simulink model "cascaded_droop_vi"  (R2021b)
settings: Solver=ode23t  StartTime=0.0  StopTime=20  RelTol=1e-3
values from neighbouring files (symbols this model uses):
  Cf_1 = 16e-6    (= 1.6e-05)    [parameters.m]
  fn = 50    [parameters.m]
  G_int = c2d(tf([wv 0],[1 wv]),Ts/2,'tustin')    [parameters.m]
  G_LPFd2 = c2d(tf([k*wn 0],[1 k*wn wn^2]),Ts/2,'tustin')    [parameters.m]
  Ilim = In    [parameters.m]
  ki_u = kp_u/Ti_u    [parameters.m]
  Kic_1 = (Rf_1)/T_i    (= 640)    [parameters.m]
  kp = delta_f/delta_P    (= 0.002)    [parameters.m]
  kp_u = Cf*w_c    [parameters.m]
  Kpc_1 = Rf_1/(exp(Rf_1/Lf_1*Ts/2)-1)    [parameters.m]
  Lf_1 = 5.6e-3    (= 0.0056)    [parameters.m]
  Lg_1 = 1e-3    (= 0.001)    [parameters.m]
  Lv = kQ/wn    [parameters.m]
  Pr = 2000    [parameters.m]
  RCf_1 = 0    [parameters.m]
  Rf_1 = 0.1    [parameters.m]
  Rg_1 = 0.08    [parameters.m]
  Rv = kQ/10    [parameters.m]
  Ts = 1/fs    (= 0.0003125)    [parameters.m]
  Ts_sim = Ts/100    (= 3.125e-06)    [parameters.m]
  Vdc = 800*sf_v    [parameters.m]
  Vn = 181*sqrt(2)*sf_v    [parameters.m]
  wn = 2*pi*fn    (= 314.159265359)    [parameters.m]
undefined symbols (not defined in the file or in its folder): DiscIntNeverNeededParam, plecs
libraries: spsVoltageMeasurementLib x15, spsCurrentMeasurementLib x12, spsabctoAlphaBetaZeroLib x10, spsThreePhaseSeriesRLCBranchLib x8, eeGeneralControl x7, spsThreePhaseVIMeasurementLib x4, spsGroundLib x3, spsThreePhaseSourceLib x2, spsDCVoltageSourceLib x2, spsEdgeDetectorLib x2, spsTriangleGeneratorLib x2, spsThreePhaseBreakerLib x2
(part 1 of 2)
settings Model: Creator=Thanh Hung Mai  LastModifiedBy=Thanh Hung Mai
settings DebuggingCC: UnconnectedInputMsg=none  UnconnectedOutputMsg=none  UnconnectedLineMsg=none
settings ModelReferenceCC: EnableRefExpFcnMdlSchedulingChecks=off
settings RTWCC: DLArmComputeVersion=20.02.1

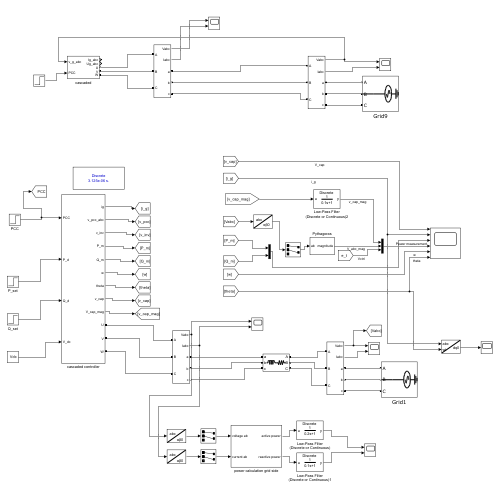
[thumbnail: Simulink's stored preview of the top-level diagram]
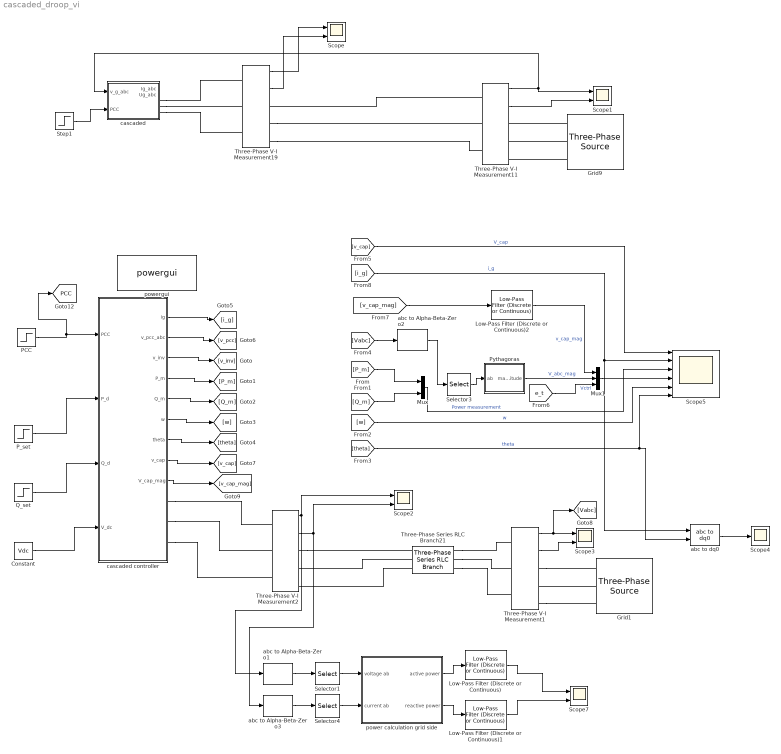
== system cascaded_droop_vi ==
  Constant : Constant  Value=Vdc
  Grid1 : spsThreePhaseSourceLib/Three-Phase Source  InternalConnection=Yg  VoltagePhases=off  Voltage=sqrt(3)*Vn/(sqrt(2))  PhaseAngle=20  Voltage_phases=[25e3 25e3 25e3]/sqrt(3)  PhaseAngles_phases=[0 -120 +120]  Frequency=50  NonIdealSource=off  SpecifyImpedance=off  Resistance=0  Inductance=0  ShortCircuitLevel=10e6  BaseVoltage=sqrt(3)*Vn/sqrt(2)  XRratio=2  BusType=swing  Pref=0  Qref=0  Prefabc=[10e3, 10e3, 10e3]  Qrefabc=[0, 0, 0]  Qmin=-inf  Qmax=inf
  Grid9 : spsThreePhaseSourceLib/Three-Phase Source  InternalConnection=Yg  VoltagePhases=off  Voltage=sqrt(3)*Vn/(sqrt(2))  PhaseAngle=0  Voltage_phases=[25e3 25e3 25e3]/sqrt(3)  PhaseAngles_phases=[0 -120 +120]  Frequency=fn  NonIdealSource=off  SpecifyImpedance=off  Resistance=0  Inductance=0  ShortCircuitLevel=10e6  BaseVoltage=sqrt(3)*Vn/sqrt(2)  XRratio=2  BusType=swing  Pref=0  Qref=0  Prefabc=[10e3, 10e3, 10e3]  Qrefabc=[0, 0, 0]  Qmin=-inf  Qmax=inf
  Low-Pass Filter (Discrete or Continuous) : eeGeneralControl/Low-Pass Filter (Discrete or Continuous)  K=1  T=0.2  B=inf  A=-inf  init_option=Inherited from block input  x0=0  Ts=-1
  Low-Pass Filter (Discrete or Continuous)1 : eeGeneralControl/Low-Pass Filter (Discrete or Continuous)  K=1  T=0.1  B=inf  A=-inf  init_option=Inherited from block input  x0=0  Ts=-1
  Low-Pass Filter (Discrete or Continuous)2 : eeGeneralControl/Low-Pass Filter (Discrete or Continuous)  K=1  T=0.1  B=inf  A=-inf  init_option=Inherited from block input  x0=0  Ts=-1
  Mux : Mux  Inputs=2
  Mux1 : Mux  Inputs=3
  PCC : Step  Time=0.4  SampleTime=Ts_sim
  P_set : Step  After=1000  SampleTime=Ts_sim
  Pythagoras : Subsystem
  Q_set : Step  Time=0  After=0  SampleTime=Ts_sim
  Scope{,1..3,7} (5 alike) : Scope  NumInputPorts=2
  Scope4 : Scope
  Scope5 : Scope  NumInputPorts=6
  Selector1 : Selector  IndexMode=Zero-based  InputPortWidth=3  IndexOptions=Index vector (dialog)  Indices=[0 1]  OutputSizes=1
  Selector3 : Selector  IndexMode=Zero-based  InputPortWidth=3  IndexOptions=Index vector (dialog)  Indices=[0 1]  OutputSizes=1
  Selector4 : Selector  IndexMode=Zero-based  InputPortWidth=3  IndexOptions=Index vector (dialog)  Indices=[0 1]  OutputSizes=1
  Step1 : Step  Time=0.5  SampleTime=0
  Three-Phase Series RLC Branch21 : spsThreePhaseSeriesRLCBranchLib/Three-Phase Series RLC Branch  LConnTagsString=A|B|C  RConnTagsString=A|B|C  BranchType=RL  Resistance=0.55  Inductance=4.39e-3  Capacitance=1e-6  Measurements=None
  Three-Phase V-I Measurement{1..2,11,19} (4 alike) : spsThreePhaseVIMeasurementLib/Three-Phase V-I Measurement  VoltageMeasurement=phase-to-ground  SetLabelV=off  LabelV=Vabc  Vpu=off  VpuLL=off  CurrentMeasurement=yes  SetLabelI=off  LabelI=Iabc  Ipu=off  Pbase=100e6  Vbase=500e3  OutputType=Complex  PhasorSimulation=off  PSBequivalent=0
  abc to Alpha-Beta-Zero1 : spsabctoAlphaBetaZeroLib/abc to Alpha-Beta-Zero
  abc to Alpha-Beta-Zero2 : spsabctoAlphaBetaZeroLib/abc to Alpha-Beta-Zero
  abc to Alpha-Beta-Zero3 : spsabctoAlphaBetaZeroLib/abc to Alpha-Beta-Zero
  abc to dq0 : spsabctodq0Lib/abc to dq0  Alignment=90 degrees behind phase A axis
  cascaded : Subsystem  VariantControl=cascaded
  cascaded controller : Subsystem  VariantControl=cascaded
  power calculation grid side : Subsystem
  powergui : spspowerguiLib/powergui  Priority=1  SimulationMode=Discrete  SampleTime=Ts_sim  frequency=60  Iterations=50  frequencyindice=50  Pbase=100e6  ErrMax=1e-4  UnitsV=kV  UnitsW=MW  buscounter=0  FunctionMessages=off  echomessages=off  EnableUseOfTLC=off  CurrentSourceSwitches=off  DisableSnubberDevices=off  DisableRonSwitches=off  DisableVfSwitches=off  DisplayEquations=off  AutomaticDiscreteSolvers=off  SolverType=Backward Euler  Interpol=off  ExternalGateDelay=off  methode=off  Ts=0  x0status=blocks  SPID=on  SwTol=0  HookPort=off  NonlinearTolerance=1e-4  nMaxIteration=100  ContinueOnMaxIteration=off  RestoreLinks=warning  ResistiveCurrentMeasurement=off  Frange=[0:2:500]  Ylog=off  Xlog=on  ShowGrid=off  save=off  variable=ZData  structure=0  ZoomFFT=off  StartTime=0.0  cycles=1  DisplayStyle=1  fundamental=60  FreqAxis=off  MaxFrequency=1000  frequencyindicesteady=1  RmsSteady=1  display=off
  tag scope: PCC=global
  wires:
  Three-Phase V-I Measurement11/1 -> cascaded/1(v_g_abc), Scope1/1
  Step1/1 -> cascaded/2(PCC)
  Three-Phase V-I Measurement19/1 -> Scope/1
  Three-Phase V-I Measurement19/2 -> Scope/2
  Three-Phase V-I Measurement11/2 -> Scope1/2
  [theta] -> abc to dq0/2, Scope5/6  "theta"
  cascaded controller/1(ig) -> [i_g]
  abc to Alpha-Beta-Zero1/1 -> Selector1/1
  [Q_m] -> Mux/2
  Q_set/1 -> cascaded controller/3(Q_d)
  Low-Pass Filter (Discrete or Continuous)/1 -> Scope7/1
  Selector1/1 -> power calculation grid side/1(voltage ab)
  Low-Pass Filter (Discrete or Continuous)1/1 -> Scope7/2
  cascaded controller/8(v_cap) -> [v_cap]
  Pythagoras/1(magnitude) -> Mux1/2  "V_abc_mag"
  Constant/1 -> cascaded controller/4(V_dc)
  [v_cap] -> Scope5/1  "V_cap"
  [P_m] -> Mux/1
  Three-Phase V-I Measurement2/1 -> abc to Alpha-Beta-Zero1/1, Scope2/1
  Three-Phase V-I Measurement2/2 -> abc to Alpha-Beta-Zero3/1, Scope2/2
  cascaded controller/9(V_cap_mag) -> [v_cap_mag]
  power calculation grid side/1(active power) -> Low-Pass Filter (Discrete or Continuous)/1
  Selector4/1 -> power calculation grid side/2(current ab)
  cascaded controller/6(w) -> [w]
  cascaded controller/4(P_m) -> [P_m]
  cascaded controller/3(v_inv) -> [v_inv]
  cascaded controller/7(theta) -> [theta]
  cascaded controller/5(Q_m) -> [Q_m]
  Low-Pass Filter (Discrete or Continuous)2/1 -> Mux1/1  "v_cap_mag"
  P_set/1 -> cascaded controller/2(P_d)
  [e_t] -> Mux1/3  "Vctrl"
  cascaded controller/2(v_pcc_abc) -> [v_pcc]
  PCC/1 -> [PCC], cascaded controller/1(PCC)
  abc to Alpha-Beta-Zero3/1 -> Selector4/1
  abc to Alpha-Beta-Zero2/1 -> Selector3/1
  Three-Phase V-I Measurement1/1 -> [Vabc], Scope3/1
  [Vabc] -> abc to Alpha-Beta-Zero2/1
  [w] -> Scope5/5  "w"
  Mux1/1 -> Scope5/4
  power calculation grid side/2(reactive power) -> Low-Pass Filter (Discrete or Continuous)1/1
  [i_g] -> abc to dq0/1, Scope5/2  "i_g"
  Selector3/1 -> Pythagoras/1(ab)
  [v_cap_mag] -> Low-Pass Filter (Discrete or Continuous)2/1
  Three-Phase V-I Measurement1/2 -> Scope3/2
  abc to dq0/1 -> Scope4/1
  Mux/1 -> Scope5/3  "Power measurement"
  connections:
  Three-Phase V-I Measurement11/LConn1 -- Three-Phase V-I Measurement19/RConn1
  cascaded/RConn3 -- Three-Phase V-I Measurement19/LConn3
  cascaded/RConn2 -- Three-Phase V-I Measurement19/LConn2
  Three-Phase V-I Measurement19/RConn3 -- Three-Phase V-I Measurement11/LConn3
  cascaded/RConn1 -- Three-Phase V-I Measurement19/LConn1
  Grid9/RConn1 -- Three-Phase V-I Measurement11/RConn1
  Three-Phase V-I Measurement19/RConn2 -- Three-Phase V-I Measurement11/LConn2
  Grid9/RConn2 -- Three-Phase V-I Measurement11/RConn2
  Grid9/RConn3 -- Three-Phase V-I Measurement11/RConn3
  Three-Phase V-I Measurement1/RConn1 -- Grid1/RConn1
  cascaded controller/RConn2 -- Three-Phase V-I Measurement2/LConn2
  Grid1/RConn2 -- Three-Phase V-I Measurement1/RConn2
  Three-Phase V-I Measurement1/RConn3 -- Grid1/RConn3
  cascaded controller/RConn1 -- Three-Phase V-I Measurement2/LConn1
  cascaded controller/RConn3 -- Three-Phase V-I Measurement2/LConn3
  Three-Phase V-I Measurement2/RConn1 -- Three-Phase Series RLC Branch21/RConn1
  Three-Phase Series RLC Branch21/RConn2 -- Three-Phase V-I Measurement2/RConn2
  Three-Phase Series RLC Branch21/RConn3 -- Three-Phase V-I Measurement2/RConn3
  Three-Phase Series RLC Branch21/LConn1 -- Three-Phase V-I Measurement1/LConn1
  Three-Phase Series RLC Branch21/LConn2 -- Three-Phase V-I Measurement1/LConn2
  Three-Phase Series RLC Branch21/LConn3 -- Three-Phase V-I Measurement1/LConn3

== system cascaded_droop_vi/Pythagoras ==
  ab : Inport
  Sqrt : Sqrt  SaturateOnIntegerOverflow=on
  Square : Math  Operator=square  SignedPower=on  RndMeth=Zero  SaturateOnIntegerOverflow=on
  Sum of Elements : Sum  Inputs=+
  magnitude : Outport  VectorParamsAs1DForOutWhenUnconnected=off
  wires:
  Sqrt/1 -> magnitude/1
  ab/1 -> Square/1
  Square/1 -> Sum of Elements/1
  Sum of Elements/1 -> Sqrt/1

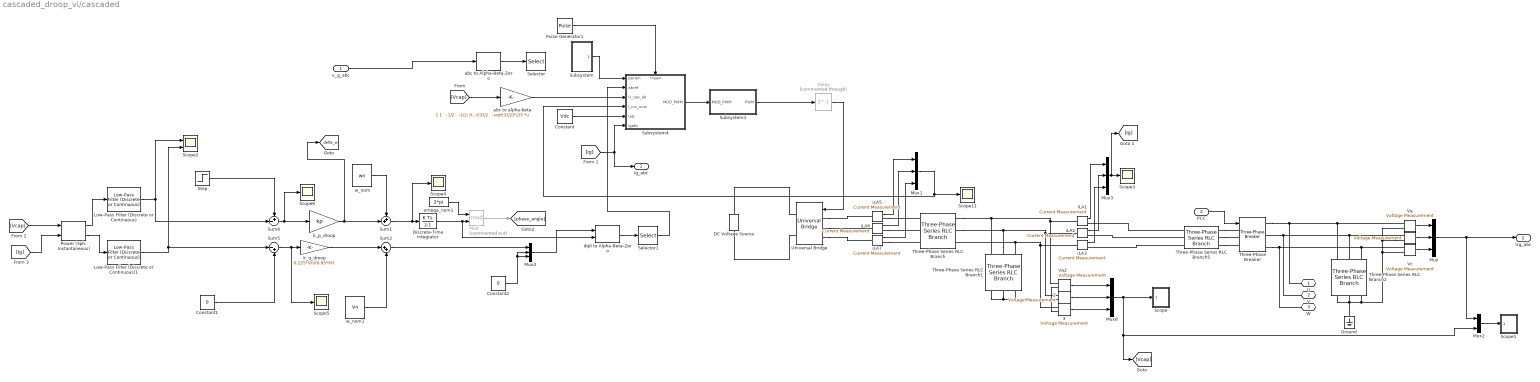
== system cascaded_droop_vi/cascaded ==
  v_g_abc : Inport
  PCC : Inport  Port=2
  "   " : spsVoltageMeasurementLib/Voltage Measurement  PhasorSimulation=off  OutputType=Complex  PSBequivalent=0
  "   2" : spsVoltageMeasurementLib/Voltage Measurement  PhasorSimulation=off  OutputType=Complex  PSBequivalent=0
  "   3" : spsVoltageMeasurementLib/Voltage Measurement  PhasorSimulation=off  OutputType=Complex  PSBequivalent=0
  Constant : Constant  Value=Vdc
  Constant1 : Constant  Value=0
  Constant2 : Constant  Value=0
  DC Voltage Source : spsDCVoltageSourceLib/DC Voltage Source  Amplitude=Vdc  Measurements=None
  Delay : Delay  Commented=through  DelayLength=1
  Discrete-Time Integrator : DiscreteIntegrator  SampleTime=-1  ICPrevOutput=DiscIntNeverNeededParam  ICPrevScaledInput=DiscIntNeverNeededParam
  Ground : spsGroundLib/Ground  LConnTagsString=a
  Low-Pass Filter (Discrete or Continuous) : eeGeneralControl/Low-Pass Filter (Discrete or Continuous)  K=1  T=0.2  B=inf  A=-inf  init_option=Inherited from block input  x0=0  Ts=-1
  Low-Pass Filter (Discrete or Continuous)1 : eeGeneralControl/Low-Pass Filter (Discrete or Continuous)  K=1  T=0.2  B=inf  A=-inf  init_option=Inherited from block input  x0=0  Ts=-1
  Mod : Math  Commented=on  Operator=mod  SaturateOnIntegerOverflow=on
  Mux{,1,3..4,8} (5 alike) : Mux  Inputs=3
  Mux2 : Mux  Inputs=2
  "Power (3ph, Instantaneous) " : spsPower3phInstantaneousLib/Power (3ph, Instantaneous)
  Pulse Generator1 : DiscretePulseGenerator  PulseType=Time based  Period=Ts/2%1/1.5e5  PulseWidth=50
  Scope : Subsystem  LoadFcn=plecs('sl', 300);  InitFcn=plecs('sl', 314);  StartFcn=plecs('sl', 308);  StopFcn=plecs('sl', 309);  mask{Settings=<binary blob, 1052 chars, not shown>}
      mask init:
      | plecs('sl', 315);
      settings: CopyFcn=plecs('sl', 303);  DeleteFcn=plecs('sl', 305);  UndoDeleteFcn=plecs('sl', 306);  PreSaveFcn=plecs('sl', 311);  NameChangeFcn=plecs('sl', 310);  DestroyFcn=plecs('sl', 307);  OpenFcn=plecs('sl', 302);  ErrorFcn=plerrorfcn
      mask Display: plot([0.1 0.9 0.9 0.1 0.1], [0.9 0.9 0.5 0.5 0.9])
  Scope1 : Subsystem  LoadFcn=plecs('sl', 300);  InitFcn=plecs('sl', 314);  StartFcn=plecs('sl', 308);  StopFcn=plecs('sl', 309);  mask{Settings=<binary blob, 1032 chars, not shown>}
      mask init:
      | plecs('sl', 315);
      settings: CopyFcn=plecs('sl', 303);  DeleteFcn=plecs('sl', 305);  UndoDeleteFcn=plecs('sl', 306);  PreSaveFcn=plecs('sl', 311);  NameChangeFcn=plecs('sl', 310);  DestroyFcn=plecs('sl', 307);  OpenFcn=plecs('sl', 302);  ErrorFcn=plerrorfcn
      mask Display: plot([0.1 0.9 0.9 0.1 0.1], [0.9 0.9 0.5 0.5 0.9])
  Scope{3..6,11} (5 alike) : Scope
  Scope2 : Scope  NumInputPorts=2
  Selector : Selector  IndexMode=Zero-based  InputPortWidth=3  IndexOptions=Index vector (dialog)  Indices=[0 1]  OutputSizes=1
  Selector1 : Selector  IndexMode=Zero-based  InputPortWidth=3  IndexOptions=Index vector (dialog)  Indices=[0 1]  OutputSizes=1
  Step : Step  After=Pr/2  SampleTime=0
  Subsystem : Subsystem
  Subsystem1 : Subsystem
  Subsystem4 : Subsystem
  Sum1 : Sum  Inputs=++|
  Sum2 : Sum  Inputs=|++
  Sum5 : Sum  Inputs=|-+
  Sum6 : Sum  Inputs=+-|
  Three-Phase Series RLC Branch : spsThreePhaseSeriesRLCBranchLib/Three-Phase Series RLC Branch  LConnTagsString=A|B|C  RConnTagsString=A|B|C  BranchType=RL  Resistance=Rf_1  Inductance=Lf_1  Capacitance=1e-6  Measurements=None
  Three-Phase Series RLC Branch1 : spsThreePhaseSeriesRLCBranchLib/Three-Phase Series RLC Branch  LConnTagsString=A|B|C  RConnTagsString=A|B|C  BranchType=RC  Resistance=RCf_1  Inductance=0.1e-3  Capacitance=Cf_1  Measurements=None
  Three-Phase Series RLC Branch2 : spsThreePhaseSeriesRLCBranchLib/Three-Phase Series RLC Branch  LConnTagsString=A|B|C  RConnTagsString=A|B|C  BranchType=R  Resistance=400e3  Inductance=0.1e-3  Capacitance=Cf_1  Measurements=None
  Three-Phase Series RLC Branch5 : spsThreePhaseSeriesRLCBranchLib/Three-Phase Series RLC Branch  LConnTagsString=A|B|C  RConnTagsString=A|B|C  BranchType=RL  Resistance=Rg_1  Inductance=Lg_1  Capacitance=1e-6  Measurements=None
  Three-Phase Breaker : spsThreePhaseBreakerLib/Three-Phase Breaker  InitialState=open  SwitchA=on  SwitchB=on  SwitchC=on  SwitchTimes=[0.1 0.9]  External=on  BreakerResistance=Ronb  SnubberResistance=Rsb  SnubberCapacitance=inf  Measurements=None
  Universal Bridge : spsUniversalBridgeLib/Universal Bridge  Arms=3  SnubberResistance=Rsi  SnubberCapacitance=inf  Device=IGBT / Diodes  Ron=Roni  Lon=0  ForwardVoltages="[  0  0  ]"  ForwardVoltage=0  GTOparameters=[ 10e-6 , 20e-6 ]  IGBTparameters=[ 1e-6 , 2e-6 ]  Measurements=None  Measurements_2=None  converterType=Rectifier
  Va : spsVoltageMeasurementLib/Voltage Measurement  PhasorSimulation=off  OutputType=Complex  PSBequivalent=0
  Va2 : spsVoltageMeasurementLib/Voltage Measurement  PhasorSimulation=off  OutputType=Complex  PSBequivalent=0
  Vc : spsVoltageMeasurementLib/Voltage Measurement  PhasorSimulation=off  OutputType=Complex  PSBequivalent=0
  abc to Alpha-Beta-Zero : spsabctoAlphaBetaZeroLib/abc to Alpha-Beta-Zero
  abc to alpha-beta : Gain  Gain="[ 1   -1/2   -1/2; 0   sqrt(3)/2   -sqrt(3)/2]*2/3"  Multiplication=Matrix(K*u) (u vector)  SaturateOnIntegerOverflow=on  OutDataTypeStr=Inherit: Same as input  ParamDataTypeStr=Inherit: Same as input
  dq0 to Alpha-Beta-Zero : spsdq0toAlphaBetaZeroLib/dq0 to Alpha-Beta-Zero  Alignment=90 degrees behind phase A axis
  iLA{1..3,5..7} (6 alike) : spsCurrentMeasurementLib/Current Measurement  PhasorSimulation=off  OutputType=Complex  PSBequivalent=0
  k_p_droop : Gain  Gain=kp
  k_q_droop : Gain  Gain=0.225*Vn/(0.95*Pr)
  omega_nom1 : Constant  Value=2*pi
  w_nom : Constant  Value=wn
  w_nom1 : Constant  Value=Vn
  U : PMIOPort  Side=Right
  V : PMIOPort  Port=2  Side=Right
  W : PMIOPort  Port=3  Side=Right
  Ig_abc : Outport  VectorParamsAs1DForOutWhenUnconnected=off
  Ug_abc : Outport  Port=2  VectorParamsAs1DForOutWhenUnconnected=off
  tag scope: delta_w=global
  wires:
  Mux2/1 -> Scope1/1(1)
  Subsystem4/1(MOD_PWM) -> Subsystem1/1(MOD_PWM)
  Mux/1 -> Mux2/1, Ug_abc/1
  Va2/1 -> Mux8/1
  iLA6/1 -> Mux1/2
  Constant/1 -> Subsystem4/5(Udc)
  Subsystem/1(param) -> Subsystem4/1(param)
  iLA3/1 -> Mux3/3
  PCC/1 -> Three-Phase Breaker/1
  Va/1 -> Mux/1
  Mux8/1 -> [Vcap], Mux2/2, Scope/1(1)
  Pulse Generator1/1 -> Subsystem4/Trigger
  iLA5/1 -> Mux1/1
  iLA2/1 -> Mux3/2
  iLA7/1 -> Mux1/3
  "   3"/1 -> Mux8/3
  "   "/1 -> Mux/2
  Mux1/1 -> Scope11/1, Subsystem4/4(I_inv_uvw)
  "   2"/1 -> Mux8/2
  Vc/1 -> Mux/3
  iLA1/1 -> Mux3/1
  Mux3/1 -> [Ig], Scope3/1
  Subsystem1/1(PWM) -> Delay/1
  Delay/1 -> Universal Bridge/1
  [Vcap] -> abc to alpha-beta/1
  [Ig] -> Ig_abc/1, Subsystem4/6(Igabc)
  [Vcap] -> "Power (3ph, Instantaneous) "/1
  [Ig] -> "Power (3ph, Instantaneous) "/2
  "Power (3ph, Instantaneous) "/1 -> Low-Pass Filter (Discrete or Continuous)/1
  "Power (3ph, Instantaneous) "/2 -> Low-Pass Filter (Discrete or Continuous)1/1
  Sum5/1 -> Scope5/1, k_q_droop/1
  w_nom1/1 -> Sum2/2
  Constant1/1 -> Sum5/2
  Sum6/1 -> Scope6/1, k_p_droop/1
  Step/1 -> Sum6/1
  w_nom/1 -> Sum1/1
  Sum2/1 -> Mux4/1
  Low-Pass Filter (Discrete or Continuous)/1 -> Sum6/2, Scope2/1
  Low-Pass Filter (Discrete or Continuous)1/1 -> Sum5/1, Scope2/2
  k_p_droop/1 -> [delta_w], Sum1/2
  Sum1/1 -> Scope4/1, Discrete-Time Integrator/1
  k_q_droop/1 -> Sum2/1
  Discrete-Time Integrator/1 -> dq0 to Alpha-Beta-Zero/2, Mod/2
  Mod/1 -> [phase_angle]
  omega_nom1/1 -> Mod/1
  abc to Alpha-Beta-Zero/1 -> Selector/1
  Mux4/1 -> dq0 to Alpha-Beta-Zero/1
  Constant2/1 -> Mux4/2, Mux4/3
  dq0 to Alpha-Beta-Zero/1 -> Selector1/1
  v_g_abc/1 -> abc to Alpha-Beta-Zero/1
  abc to alpha-beta/1 -> Subsystem4/3(U_cap_ab)
  Selector1/1 -> Subsystem4/2(abref)
  connections:
  "   "/LConn2 -- Ground/LConn1 -- Three-Phase Series RLC Branch2/RConn1 -- Three-Phase Series RLC Branch2/RConn2 -- Three-Phase Series RLC Branch2/RConn3 -- Vc/LConn2 -- Va/LConn2
  Three-Phase Series RLC Branch5/LConn1 -- Three-Phase Breaker/LConn1
  Three-Phase Breaker/RConn1 -- Three-Phase Series RLC Branch2/LConn1 -- Va/LConn1 -- U/RConn1
  DC Voltage Source/RConn1 -- Universal Bridge/RConn1
  iLA7/RConn1 -- Three-Phase Series RLC Branch/LConn3
  Va2/LConn2 -- Three-Phase Series RLC Branch1/RConn1 -- Three-Phase Series RLC Branch1/RConn2 -- Three-Phase Series RLC Branch1/RConn3 -- "   3"/LConn2 -- "   2"/LConn2
  Universal Bridge/LConn2 -- iLA6/LConn1
  iLA5/RConn1 -- Three-Phase Series RLC Branch/LConn1
  Three-Phase Series RLC Branch1/LConn2 -- Three-Phase Series RLC Branch/RConn2 -- iLA2/LConn1 -- "   2"/LConn1
  Three-Phase Series RLC Branch5/RConn1 -- iLA1/RConn1
  iLA6/RConn1 -- Three-Phase Series RLC Branch/LConn2
  Universal Bridge/LConn3 -- iLA7/LConn1
  Three-Phase Series RLC Branch5/LConn3 -- Three-Phase Breaker/LConn3
  Three-Phase Series RLC Branch/RConn3 -- Three-Phase Series RLC Branch1/LConn3 -- iLA3/LConn1 -- "   3"/LConn1
  "   "/LConn1 -- Three-Phase Series RLC Branch2/LConn2 -- Three-Phase Breaker/RConn2 -- V/RConn1
  DC Voltage Source/LConn1 -- Universal Bridge/RConn2
  Universal Bridge/LConn1 -- iLA5/LConn1
  Three-Phase Series RLC Branch5/LConn2 -- Three-Phase Breaker/LConn2
  Three-Phase Series RLC Branch5/RConn3 -- iLA3/RConn1
  Three-Phase Series RLC Branch/RConn1 -- Three-Phase Series RLC Branch1/LConn1 -- iLA1/LConn1 -- Va2/LConn1
  Three-Phase Breaker/RConn3 -- Three-Phase Series RLC Branch2/LConn3 -- Vc/LConn1 -- W/RConn1
  Three-Phase Series RLC Branch5/RConn2 -- iLA2/RConn1

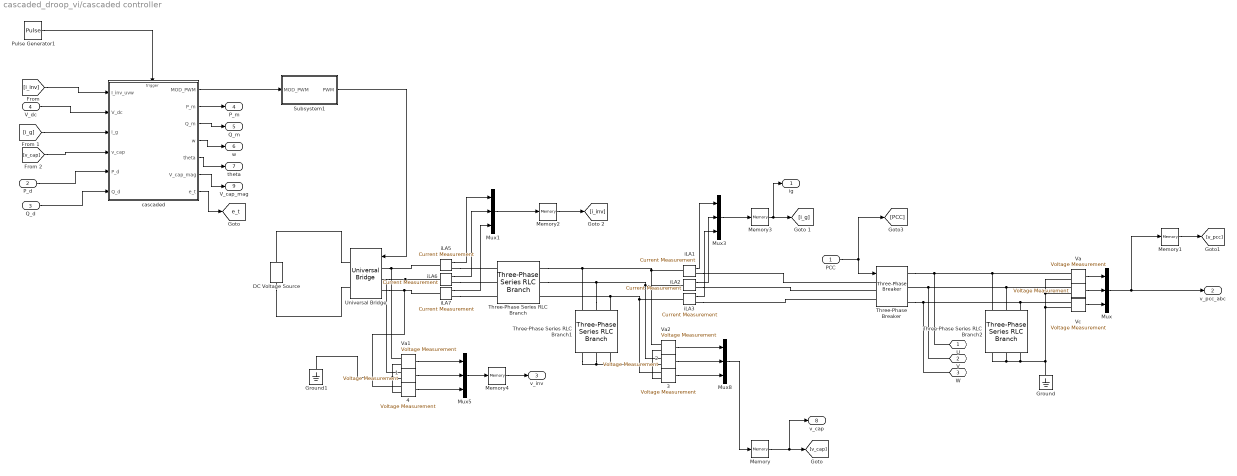
== system cascaded_droop_vi/cascaded controller ==
  PCC : Inport
  P_d : Inport  Port=2
  Q_d : Inport  Port=3
  V_dc : Inport  Port=4
     {,1..4} (5 alike) : spsVoltageMeasurementLib/Voltage Measurement  PhasorSimulation=off  OutputType=Complex  PSBequivalent=0
  DC Voltage Source : spsDCVoltageSourceLib/DC Voltage Source  Amplitude=Vdc  Measurements=None
  Ground : spsGroundLib/Ground  LConnTagsString=a
  Ground1 : spsGroundLib/Ground  LConnTagsString=a
  Memory{,1..4} (5 alike) : Memory
  Mux{,1,3,5,8} (5 alike) : Mux  Inputs=3
  Pulse Generator1 : DiscretePulseGenerator  PulseType=Time based  Period=Ts/2%1/1.5e5  PulseWidth=50
  Subsystem1 : Subsystem
  Three-Phase Series RLC Branch : spsThreePhaseSeriesRLCBranchLib/Three-Phase Series RLC Branch  LConnTagsString=A|B|C  RConnTagsString=A|B|C  BranchType=RL  Resistance=Rf_1  Inductance=Lf_1  Capacitance=1e-6  Measurements=None
  Three-Phase Series RLC Branch1 : spsThreePhaseSeriesRLCBranchLib/Three-Phase Series RLC Branch  LConnTagsString=A|B|C  RConnTagsString=A|B|C  BranchType=RC  Resistance=RCf_1  Inductance=0.1e-3  Capacitance=Cf_1  Measurements=None
  Three-Phase Series RLC Branch2 : spsThreePhaseSeriesRLCBranchLib/Three-Phase Series RLC Branch  LConnTagsString=A|B|C  RConnTagsString=A|B|C  BranchType=R  Resistance=400e3  Inductance=0.1e-3  Capacitance=Cf_1  Measurements=None
  Three-Phase Breaker : spsThreePhaseBreakerLib/Three-Phase Breaker  InitialState=open  SwitchA=on  SwitchB=on  SwitchC=on  SwitchTimes=[0.1 0.9]  External=on  BreakerResistance=Ronb  SnubberResistance=Rsb  SnubberCapacitance=inf  Measurements=None
  Universal Bridge : spsUniversalBridgeLib/Universal Bridge  Arms=3  SnubberResistance=Rsi  SnubberCapacitance=inf  Device=IGBT / Diodes  Ron=Roni  Lon=0  ForwardVoltages="[  0  0  ]"  ForwardVoltage=0  GTOparameters=[ 10e-6 , 20e-6 ]  IGBTparameters=[ 1e-6 , 2e-6 ]  Measurements=None  Measurements_2=None  converterType=Rectifier
  Va : spsVoltageMeasurementLib/Voltage Measurement  PhasorSimulation=off  OutputType=Complex  PSBequivalent=0
  Va1 : spsVoltageMeasurementLib/Voltage Measurement  PhasorSimulation=off  OutputType=Complex  PSBequivalent=0
  Va2 : spsVoltageMeasurementLib/Voltage Measurement  PhasorSimulation=off  OutputType=Complex  PSBequivalent=0
  Vc : spsVoltageMeasurementLib/Voltage Measurement  PhasorSimulation=off  OutputType=Complex  PSBequivalent=0
  cascaded : Subsystem
  iLA{1..3,5..7} (6 alike) : spsCurrentMeasurementLib/Current Measurement  PhasorSimulation=off  OutputType=Complex  PSBequivalent=0
  U : PMIOPort  Side=Right
  V : PMIOPort  Port=2  Side=Right
  W : PMIOPort  Port=3  Side=Right
  ig : Outport  VectorParamsAs1DForOutWhenUnconnected=off
  v_pcc_abc : Outport  Port=2  VectorParamsAs1DForOutWhenUnconnected=off
  v_inv : Outport  Port=3  VectorParamsAs1DForOutWhenUnconnected=off
  P_m : Outport  Port=4
  Q_m : Outport  Port=5
  w : Outport  Port=6
  theta : Outport  Port=7
  v_cap : Outport  Port=8  VectorParamsAs1DForOutWhenUnconnected=off
  V_cap_mag : Outport  Port=9  VectorParamsAs1DForOutWhenUnconnected=off
  tag scope: e_t=global
  wires:
  cascaded/1(MOD_PWM) -> Subsystem1/1(MOD_PWM)
  Mux/1 -> Memory1/1, v_pcc_abc/1
  Va2/1 -> Mux8/1
  iLA6/1 -> Mux1/2
  V_dc/1 -> cascaded/2(V_dc)
  iLA3/1 -> Mux3/3
  PCC/1 -> [PCC], Three-Phase Breaker/1
  Va/1 -> Mux/1
  iLA5/1 -> Mux1/1
  iLA2/1 -> Mux3/2
  iLA7/1 -> Mux1/3
  "   3"/1 -> Mux8/3
  "   "/1 -> Mux/2
  "   2"/1 -> Mux8/2
  Vc/1 -> Mux/3
  iLA1/1 -> Mux3/1
  Mux3/1 -> Memory3/1
  Subsystem1/1(PWM) -> Universal Bridge/1
  [i_g] -> cascaded/3(i_g)
  "   4"/1 -> Mux5/3
  Va1/1 -> Mux5/1
  "   1"/1 -> Mux5/2
  Memory/1 -> v_cap/1, [v_cap]
  Memory1/1 -> [v_pcc]
  Mux1/1 -> Memory2/1
  Memory2/1 -> [i_inv]
  [i_inv] -> cascaded/1(I_inv_uvw)
  [v_cap] -> cascaded/4(v_cap)
  Memory3/1 -> ig/1, [i_g]
  Mux5/1 -> Memory4/1
  Memory4/1 -> v_inv/1
  cascaded/5(theta) -> theta/1
  cascaded/4(w) -> w/1
  cascaded/3(Q_m) -> Q_m/1
  cascaded/2(P_m) -> P_m/1
  Q_d/1 -> cascaded/6(Q_d)
  P_d/1 -> cascaded/5(P_d)
  cascaded/6(V_cap_mag) -> V_cap_mag/1
  Mux8/1 -> Memory/1
  cascaded/7(e_t) -> [e_t]
  Pulse Generator1/1 -> cascaded/Trigger
  connections:
  Three-Phase Series RLC Branch2/RConn2 -- "   "/LConn2 -- Va/LConn2 -- Vc/LConn2 -- Ground/LConn1 -- Three-Phase Series RLC Branch2/RConn3 -- Three-Phase Series RLC Branch2/RConn1
  iLA1/RConn1 -- Three-Phase Breaker/LConn1
  Three-Phase Breaker/RConn1 -- U/RConn1 -- Three-Phase Series RLC Branch2/LConn1 -- Va/LConn1
  DC Voltage Source/RConn1 -- Universal Bridge/RConn1
  iLA7/RConn1 -- Three-Phase Series RLC Branch/LConn3
  Va2/LConn2 -- Three-Phase Series RLC Branch1/RConn1 -- Three-Phase Series RLC Branch1/RConn2 -- Three-Phase Series RLC Branch1/RConn3 -- "   3"/LConn2 -- "   2"/LConn2
  Universal Bridge/LConn2 -- "   1"/LConn1 -- iLA6/LConn1
  iLA5/RConn1 -- Three-Phase Series RLC Branch/LConn1
  Three-Phase Series RLC Branch1/LConn2 -- Three-Phase Series RLC Branch/RConn2 -- iLA2/LConn1 -- "   2"/LConn1
  iLA6/RConn1 -- Three-Phase Series RLC Branch/LConn2
  Universal Bridge/LConn3 -- "   4"/LConn1 -- iLA7/LConn1
  iLA3/RConn1 -- Three-Phase Breaker/LConn3
  Three-Phase Series RLC Branch/RConn3 -- Three-Phase Series RLC Branch1/LConn3 -- iLA3/LConn1 -- "   3"/LConn1
  "   "/LConn1 -- Three-Phase Series RLC Branch2/LConn2 -- V/RConn1 -- Three-Phase Breaker/RConn2
  DC Voltage Source/LConn1 -- Universal Bridge/RConn2
  Universal Bridge/LConn1 -- Va1/LConn1 -- iLA5/LConn1
  iLA2/RConn1 -- Three-Phase Breaker/LConn2
  Three-Phase Series RLC Branch/RConn1 -- Three-Phase Series RLC Branch1/LConn1 -- iLA1/LConn1 -- Va2/LConn1
  Three-Phase Breaker/RConn3 -- Three-Phase Series RLC Branch2/LConn3 -- Vc/LConn1 -- W/RConn1
  Va1/LConn2 -- Ground1/LConn1 -- "   4"/LConn2 -- "   1"/LConn2

== system cascaded_droop_vi/power calculation grid side ==
  voltage ab : Inport
  current ab : Inport  Port=2
  Demux : Demux  Outputs=2
  Demux1 : Demux  Outputs=2
  Gain1 : Gain  Gain=3/2
  Gain3 : Gain  Gain=3/2
  Product{1,4..6} (4 alike) : Product  InputSameDT=on  SaturateOnIntegerOverflow=on  OutDataTypeStr=Inherit: Same as first input
  Sum2 : Sum  Inputs=+-
  Sum3 : Sum
  abc to alpha-beta3 : Subsystem
  active power : Outport
  reactive power : Outport  Port=2
  wires:
  Product6/1 -> Sum2/2
  Product1/1 -> Sum2/1
  Sum2/1 -> Gain1/1
  Gain3/1 -> active power/1
  Product5/1 -> Sum3/2
  Demux1/2 -> Product5/2, Product6/2
  Demux/2 -> Product5/1, Product1/1
  Product4/1 -> Sum3/1
  Demux1/1 -> Product4/2, Product1/2
  Demux/1 -> Product6/1, Product4/1
  Sum3/1 -> Gain3/1
  Gain1/1 -> reactive power/1
  current ab/1 -> Demux1/1
  voltage ab/1 -> Demux/1

== system cascaded_droop_vi/cascaded/Scope ==
  1 : Inport
  " 1 " : DataTypeConversion  SaturateOnIntegerOverflow=on  RndMeth=Zero
  " InputMux " : Mux  Inputs=1
  " S-Function " : S-Function  FunctionName=plecs  SFunctionDeploymentMode=off  EnableBusSupport=off
  wires:
  " 1 "/1 -> " InputMux "/1
  1/1 -> " 1 "/1
  " InputMux "/1 -> " S-Function "/1

== system cascaded_droop_vi/cascaded/Scope1 ==
  1 : Inport
  " 1 " : DataTypeConversion  SaturateOnIntegerOverflow=on  RndMeth=Zero
  " InputMux " : Mux  Inputs=1
  " S-Function " : S-Function  FunctionName=plecs  SFunctionDeploymentMode=off  EnableBusSupport=off
  wires:
  " InputMux "/1 -> " S-Function "/1
  1/1 -> " 1 "/1
  " 1 "/1 -> " InputMux "/1

== system cascaded_droop_vi/cascaded/Subsystem ==
  1/kp_i : Constant  Value=1/Kpc_1
  1/kp_u : Constant  Value=1/kp_u
  Bus Creator : BusCreator  Inputs=11
  E1 : Constant  Value=wn*Lf_1
  E2 : Constant  Value=Cf_1*wn
  Isat : Constant  Value=Ilim
  g_ff_i : Constant
  g_ff_v : Constant
  ki_i*Ts/2 : Constant  Value=Kic_1
  ki_u*Ts/2 : Constant  Value=ki_u
  kp_i : Constant  Value=Kpc_1
  kp_u : Constant  Value=kp_u
  param : Outport  VectorParamsAs1DForOutWhenUnconnected=off
  wires:
  Bus Creator/1 -> param/1
  g_ff_v/1 -> Bus Creator/11  "g_ff_v"
  g_ff_i/1 -> Bus Creator/10  "g_ff_i"
  Isat/1 -> Bus Creator/9  "Isat"
  E2/1 -> Bus Creator/8  "E2"
  1/kp_u/1 -> Bus Creator/7  "1/kp_u"
  ki_u*Ts/2/1 -> Bus Creator/6  "ki_u"
  kp_u/1 -> Bus Creator/5  "kp_u"
  E1/1 -> Bus Creator/4  "E1"
  1/kp_i/1 -> Bus Creator/3  "1/kp_i"
  ki_i*Ts/2/1 -> Bus Creator/2  "ki_i"
  kp_i/1 -> Bus Creator/1  "kp_i"

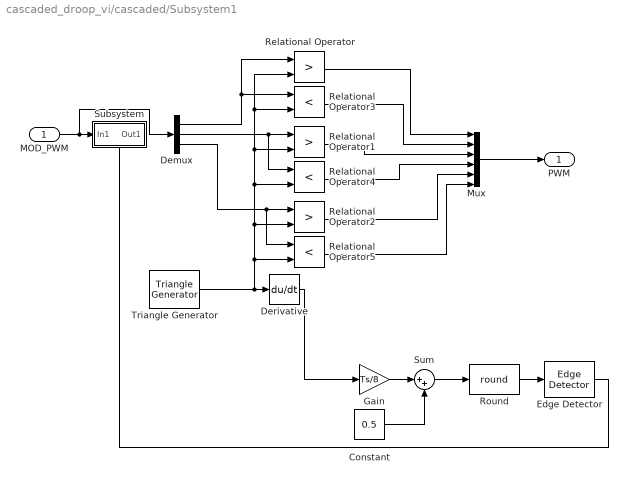
== system cascaded_droop_vi/cascaded/Subsystem1 ==
  MOD_PWM : Inport
  Constant : Constant  Value=0.5
  Demux : Demux  Outputs=3
  Derivative : Derivative
  Edge Detector : spsEdgeDetectorLib/Edge Detector  model=Either  ic=0  Ts=0
  Gain : Gain  Gain=Ts/8
  Mux : Mux  Inputs=6
  Relational Operator : RelationalOperator  Operator=>  OutDataTypeStr=boolean  RndMeth=Simplest
  Relational Operator1 : RelationalOperator  Operator=>  OutDataTypeStr=boolean  RndMeth=Simplest
  Relational Operator2 : RelationalOperator  Operator=>  OutDataTypeStr=boolean  RndMeth=Simplest
  Relational Operator3 : RelationalOperator  Operator=<  OutDataTypeStr=boolean  RndMeth=Simplest
  Relational Operator4 : RelationalOperator  Operator=<  OutDataTypeStr=boolean  RndMeth=Simplest
  Relational Operator5 : RelationalOperator  Operator=<  OutDataTypeStr=boolean  RndMeth=Simplest
  Round : Rounding  Operator=round
  Subsystem : Subsystem
  Sum : Sum  Inputs=|++
  Triangle Generator : spsTriangleGeneratorLib/Triangle Generator  Freq=fs  Phase=0  Ts=0
  PWM : Outport  VectorParamsAs1DForOutWhenUnconnected=off
  wires:
  Derivative/1 -> Gain/1
  Round/1 -> Edge Detector/1
  Sum/1 -> Round/1
  Constant/1 -> Sum/2
  Gain/1 -> Sum/1
  Relational Operator5/1 -> Mux/6
  Relational Operator2/1 -> Mux/5
  Relational Operator4/1 -> Mux/4
  Relational Operator1/1 -> Mux/3
  Relational Operator3/1 -> Mux/2
  Relational Operator/1 -> Mux/1
  Demux/3 -> Relational Operator2/1, Relational Operator5/1
  Demux/2 -> Relational Operator1/1, Relational Operator4/1
  Mux/1 -> PWM/1
  Demux/1 -> Relational Operator/1, Relational Operator3/1
  Triangle Generator/1 -> Relational Operator/2, Relational Operator3/2, Relational Operator1/2, Relational Operator4/2, Relational Operator2/2, Relational Operator5/2, Derivative/1
  Edge Detector/1 -> Subsystem/Trigger
  MOD_PWM/1 -> Demux/1, Subsystem/1(In1)

== system cascaded_droop_vi/cascaded/Subsystem4 ==
  param : Inport
  abref : Inport  Port=2
  U_cap_ab : Inport  Port=3
  I_inv_uvw : Inport  Port=4
  Udc : Inport  Port=5
  Igabc : Inport  Port=6
  Trigger : TriggerPort  VariantControl=Variant  PortDimensions=1
  Constant : Constant  Value=-2/9
  Subtract1 : Sum  Inputs=+-
  THI : Subsystem
  Virtual impedance1 : Subsystem
  abc to alpha-beta1 : Gain  Gain="[ 1   -1/2   -1/2; 0   sqrt(3)/2   -sqrt(3)/2]*2/3"  Multiplication=Matrix(K*u) (u vector)  SaturateOnIntegerOverflow=on  OutDataTypeStr=Inherit: Same as input  ParamDataTypeStr=Inherit: Same as input
  abc to alpha-beta2 : Gain  Gain="[ 1   -1/2   -1/2; 0   sqrt(3)/2   -sqrt(3)/2]*2/3"  Multiplication=Matrix(K*u) (u vector)  SaturateOnIntegerOverflow=on  OutDataTypeStr=Inherit: Same as input  ParamDataTypeStr=Inherit: Same as input
  alpha-beta to abc : Gain  Gain="[ 1   0; -1/2  sqrt(3)/2; -1/2  -sqrt(3)/2]"  Multiplication=Matrix(K*u) (u vector)  SaturateOnIntegerOverflow=on  OutDataTypeStr=Inherit: Same as input  ParamDataTypeStr=Inherit: Same as input
  current : Subsystem  VariantControl=PR
  voltage : Subsystem  VariantControl=PR
  MOD_PWM : Outport  VectorParamsAs1DForOutWhenUnconnected=off
  wires:
  Subtract1/1 -> voltage/2(U_ab_ref)
  Virtual impedance1/1(U_Lv_ab) -> Subtract1/2
  abc to alpha-beta1/1 -> Virtual impedance1/1(Ig_ab), voltage/4(Ig_ab)
  Igabc/1 -> abc to alpha-beta1/1
  param/1 -> current/1(param), voltage/1(param)
  I_inv_uvw/1 -> abc to alpha-beta2/1
  Udc/1 -> current/5(Udc)
  Constant/1 -> THI/1(THI gain)
  alpha-beta to abc/1 -> THI/2(abc)
  THI/1(abc_out) -> MOD_PWM/1
  U_cap_ab/1 -> voltage/3(U_ab), current/4(U_ab)
  abref/1 -> Subtract1/1
  voltage/1(I_ab_ref) -> current/2(I_ab_ref)
  abc to alpha-beta2/1 -> current/3(I_ab)
  current/1(U_ab_inv) -> THI/3(ab), alpha-beta to abc/1

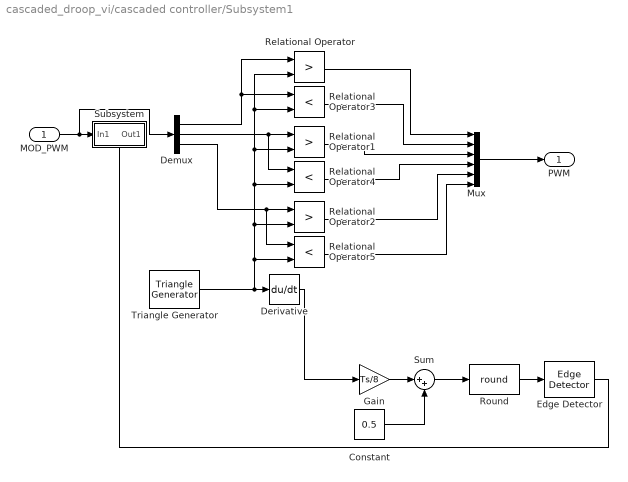
== system cascaded_droop_vi/cascaded controller/Subsystem1 ==
  MOD_PWM : Inport
  Constant : Constant  Value=0.5
  Demux : Demux  Outputs=3
  Derivative : Derivative
  Edge Detector : spsEdgeDetectorLib/Edge Detector  model=Either  ic=0  Ts=0
  Gain : Gain  Gain=Ts/8
  Mux : Mux  Inputs=6
  Relational Operator : RelationalOperator  Operator=>  OutDataTypeStr=boolean  RndMeth=Simplest
  Relational Operator1 : RelationalOperator  Operator=>  OutDataTypeStr=boolean  RndMeth=Simplest
  Relational Operator2 : RelationalOperator  Operator=>  OutDataTypeStr=boolean  RndMeth=Simplest
  Relational Operator3 : RelationalOperator  Operator=<  OutDataTypeStr=boolean  RndMeth=Simplest
  Relational Operator4 : RelationalOperator  Operator=<  OutDataTypeStr=boolean  RndMeth=Simplest
  Relational Operator5 : RelationalOperator  Operator=<  OutDataTypeStr=boolean  RndMeth=Simplest
  Round : Rounding  Operator=round
  Subsystem : Subsystem
  Sum : Sum  Inputs=|++
  Triangle Generator : spsTriangleGeneratorLib/Triangle Generator  Freq=fs  Phase=0  Ts=0
  PWM : Outport  VectorParamsAs1DForOutWhenUnconnected=off
  wires:
  Derivative/1 -> Gain/1
  Round/1 -> Edge Detector/1
  Sum/1 -> Round/1
  Constant/1 -> Sum/2
  Gain/1 -> Sum/1
  Relational Operator5/1 -> Mux/6
  Relational Operator2/1 -> Mux/5
  Relational Operator4/1 -> Mux/4
  Relational Operator1/1 -> Mux/3
  Relational Operator3/1 -> Mux/2
  Relational Operator/1 -> Mux/1
  Demux/3 -> Relational Operator2/1, Relational Operator5/1
  Demux/2 -> Relational Operator1/1, Relational Operator4/1
  Mux/1 -> PWM/1
  Demux/1 -> Relational Operator/1, Relational Operator3/1
  Triangle Generator/1 -> Relational Operator/2, Relational Operator3/2, Relational Operator1/2, Relational Operator4/2, Relational Operator2/2, Relational Operator5/2, Derivative/1
  Edge Detector/1 -> Subsystem/Trigger
  MOD_PWM/1 -> Demux/1, Subsystem/1(In1)

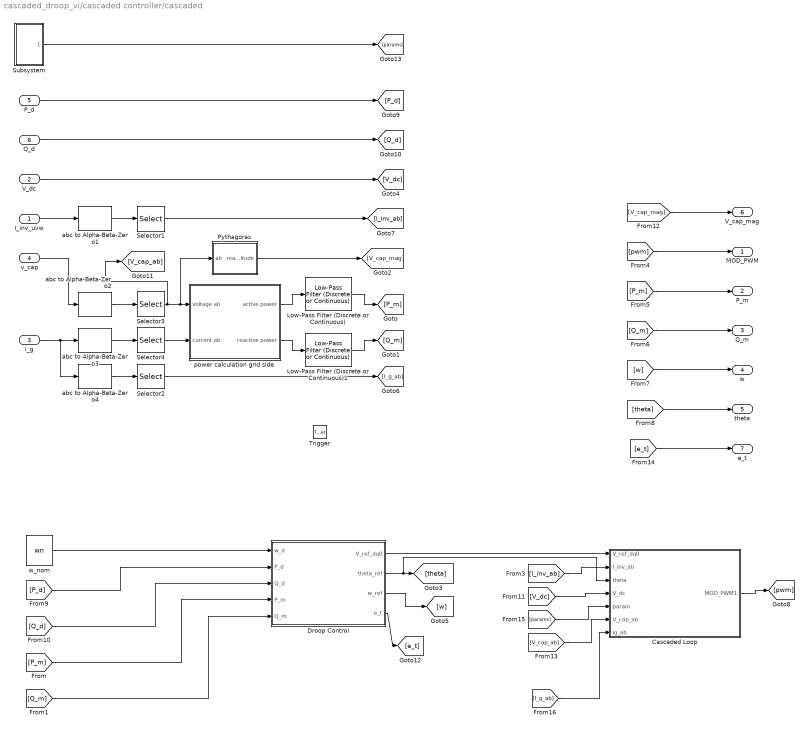
== system cascaded_droop_vi/cascaded controller/cascaded ==
  I_inv_uvw : Inport
  V_dc : Inport  Port=2
  i_g : Inport  Port=3
  v_cap : Inport  Port=4
  P_d : Inport  Port=5
  Q_d : Inport  Port=6
  Trigger : TriggerPort  VariantControl=(inherit)  PortDimensions=1
  Cascaded Loop : Subsystem
  Droop Control : Subsystem
  Low-Pass Filter (Discrete or Continuous) : eeGeneralControl/Low-Pass Filter (Discrete or Continuous)  K=1  T=0.1  B=inf  A=-inf  init_option=Inherited from block input  x0=0  Ts=-1
  Low-Pass Filter (Discrete or Continuous)1 : eeGeneralControl/Low-Pass Filter (Discrete or Continuous)  K=1  T=0.1  B=inf  A=-inf  init_option=Inherited from block input  x0=0  Ts=-1
  Pythagoras : Subsystem
  Selector{1..4} (4 alike) : Selector  IndexMode=Zero-based  InputPortWidth=3  IndexOptions=Index vector (dialog)  Indices=[0 1]  OutputSizes=1
  Subsystem : Subsystem
  abc to Alpha-Beta-Zero{1..4} (4 alike) : spsabctoAlphaBetaZeroLib/abc to Alpha-Beta-Zero
  power calculation grid side : Subsystem
  w_nom : Constant  Value=wn
  MOD_PWM : Outport  VectorParamsAs1DForOutWhenUnconnected=off
  P_m : Outport  Port=2  VectorParamsAs1DForOutWhenUnconnected=off
  Q_m : Outport  Port=3  VectorParamsAs1DForOutWhenUnconnected=off
  w : Outport  Port=4  VectorParamsAs1DForOutWhenUnconnected=off
  theta : Outport  Port=5  VectorParamsAs1DForOutWhenUnconnected=off
  V_cap_mag : Outport  Port=6  VectorParamsAs1DForOutWhenUnconnected=off
  e_t : Outport  Port=7  VectorParamsAs1DForOutWhenUnconnected=off
  wires:
  abc to Alpha-Beta-Zero2/1 -> Selector3/1
  v_cap/1 -> abc to Alpha-Beta-Zero2/1
  abc to Alpha-Beta-Zero3/1 -> Selector4/1
  i_g/1 -> abc to Alpha-Beta-Zero4/1, abc to Alpha-Beta-Zero3/1
  Pythagoras/1(magnitude) -> [V_cap_mag]
  w_nom/1 -> Droop Control/1(w_d)
  [P_d] -> Droop Control/2(P_d)
  [P_m] -> Droop Control/4(P_m)
  [Q_m] -> Droop Control/5(Q_m)
  [Q_d] -> Droop Control/3(Q_d)
  Droop Control/2(theta_ref) -> Cascaded Loop/3(theta), [theta]
  Droop Control/3(w_ref) -> [w]
  I_inv_uvw/1 -> abc to Alpha-Beta-Zero1/1
  abc to Alpha-Beta-Zero1/1 -> Selector1/1
  V_dc/1 -> [V_dc]
  abc to Alpha-Beta-Zero4/1 -> Selector2/1
  Selector2/1 -> [I_g_ab]
  [I_inv_ab] -> Cascaded Loop/2(I_inv_ab)
  Selector1/1 -> [I_inv_ab]
  Cascaded Loop/1(MOD_PWM1) -> [pwm]
  [pwm] -> MOD_PWM/1
  [P_m] -> P_m/1
  [Q_m] -> Q_m/1
  [w] -> w/1
  [theta] -> theta/1
  P_d/1 -> [P_d]
  Q_d/1 -> [Q_d]
  [V_dc] -> Cascaded Loop/4(V_dc)
  Selector3/1 -> [V_cap_ab], Pythagoras/1(ab), power calculation grid side/1(voltage ab)
  Selector4/1 -> power calculation grid side/2(current ab)
  power calculation grid side/1(active power) -> Low-Pass Filter (Discrete or Continuous)/1
  Low-Pass Filter (Discrete or Continuous)/1 -> [P_m]
  power calculation grid side/2(reactive power) -> Low-Pass Filter (Discrete or Continuous)1/1
  Low-Pass Filter (Discrete or Continuous)1/1 -> [Q_m]
  [V_cap_mag] -> V_cap_mag/1
  [V_cap_ab] -> Cascaded Loop/6(V_cap_ab)
  Droop Control/4(e_t) -> [e_t]
  [e_t] -> e_t/1
  Subsystem/1(param) -> [params]
  [params] -> Cascaded Loop/5(param)
  [I_g_ab] -> Cascaded Loop/7(ig_ab)
  Droop Control/1(V_ref_dq0) -> Cascaded Loop/1(V_ref_dq0)

== system cascaded_droop_vi/power calculation grid side/abc to alpha-beta3 ==
  abc : Inport
  Demux : Demux  Outputs=3
  Terminator1 : Terminator
  abc to Alpha-Beta-Zero : spsabctoAlphaBetaZeroLib/abc to Alpha-Beta-Zero
  alpha : Outport
  beta : Outport  Port=2
  wires:
  abc to Alpha-Beta-Zero/1 -> Demux/1
  abc/1 -> abc to Alpha-Beta-Zero/1
  Demux/3 -> Terminator1/1
  Demux/2 -> beta/1
  Demux/1 -> alpha/1

== system cascaded_droop_vi/cascaded/Subsystem1/Subsystem ==
  In1 : Inport
  Trigger : TriggerPort  VariantControl=Variant  PortDimensions=1
  Out1 : Outport  VectorParamsAs1DForOutWhenUnconnected=off
  wires:
  In1/1 -> Out1/1

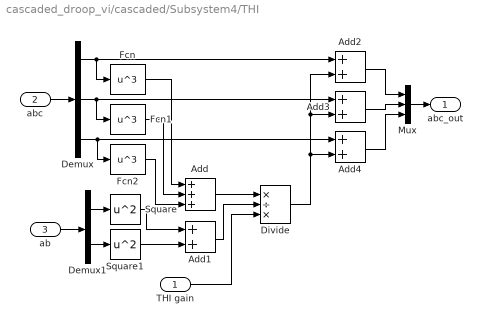
== system cascaded_droop_vi/cascaded/Subsystem4/THI ==
  THI gain : Inport
  abc : Inport  Port=2
  ab : Inport  Port=3
  Add : Sum  Inputs=+++
  Add{1..4} (4 alike) : Sum
  Demux : Demux  Outputs=3
  Demux1 : Demux  Outputs=2
  Divide : Product  Inputs=*/*
  Fcn : Fcn  Expr=u^3
  Fcn1 : Fcn  Expr=u^3
  Fcn2 : Fcn  Expr=u^3
  Mux : Mux  Inputs=3
  Square : Math  Operator=square  SignedPower=on  RndMeth=Zero  SaturateOnIntegerOverflow=on
  Square1 : Math  Operator=square  SignedPower=on  RndMeth=Zero  SaturateOnIntegerOverflow=on
  abc_out : Outport  VectorParamsAs1DForOutWhenUnconnected=off
  wires:
  Demux/2 -> Add3/1, Fcn1/1
  Fcn2/1 -> Add/3
  Fcn1/1 -> Add/2
  Fcn/1 -> Add/1
  Mux/1 -> abc_out/1
  Add4/1 -> Mux/3
  Add2/1 -> Mux/1
  Add3/1 -> Mux/2
  Divide/1 -> Add4/2, Add3/2, Add2/2
  THI gain/1 -> Divide/3
  Add1/1 -> Divide/2
  Add/1 -> Divide/1
  Square1/1 -> Add1/2
  Square/1 -> Add1/1
  Demux1/2 -> Square1/1
  Demux1/1 -> Square/1
  ab/1 -> Demux1/1
  Demux/1 -> Fcn/1, Add2/1
  Demux/3 -> Add4/1, Fcn2/1
  abc/1 -> Demux/1

== system cascaded_droop_vi/cascaded/Subsystem4/Virtual impedance1 ==
  Ig_ab : Inport
  Discrete Transfer Fcn2 : DiscreteTransferFcn  Numerator=G_int.num{1}  Denominator=G_int.den{1}
  Gain1 : Gain  Gain=Rv
  Gain2 : Gain  Gain=Lv
  Sum3 : Sum  Inputs=|++
  U_Lv_ab : Outport  VectorParamsAs1DForOutWhenUnconnected=off
  wires:
  Sum3/1 -> U_Lv_ab/1
  Gain1/1 -> Sum3/2
  Gain2/1 -> Sum3/1
  Ig_ab/1 -> Discrete Transfer Fcn2/1, Gain1/1
  Discrete Transfer Fcn2/1 -> Gain2/1

== system cascaded_droop_vi/cascaded/Subsystem4/current ==
  param : Inport
  I_ab_ref : Inport  Port=2
  I_ab : Inport  Port=3
  U_ab : Inport  Port=4
  Udc : Inport  Port=5
  Bus Selector : BusSelector  OutputSignals=E1,g_ff_v
  Delay : Delay  DelayLength=1  InitialCondition=0
  Discrete Transfer Fcn : DiscreteTransferFcn  Numerator=G_LPFd2.num{1}  Denominator=G_LPFd2.den{1}
  Divide : Product  Inputs=*/
  Gain : Gain  Gain=1/2
  Subtract : Sum  Inputs=+-
  Subtract1 : Sum  Inputs=+-
  Voltage_lim : Subsystem
  control_ab : Subsystem
  voltage_FF : Subsystem
  U_ab_inv : Outport  VectorParamsAs1DForOutWhenUnconnected=off
  wires:
  Discrete Transfer Fcn/1 -> voltage_FF/2(b)
  voltage_FF/1(ab_out) -> Voltage_lim/1(ab_in), Subtract/1
  Delay/1 -> control_ab/3(awr)
  Gain/1 -> Divide/2
  Divide/1 -> U_ab_inv/1
  Udc/1 -> Voltage_lim/2(Vdc), Gain/1
  U_ab/1 -> Discrete Transfer Fcn/1
  Subtract/1 -> Delay/1
  Bus Selector/2 -> voltage_FF/3(g_FF)  "<g_ff_v>"
  I_ab/1 -> Subtract1/2
  Subtract1/1 -> control_ab/1(in_ab)
  control_ab/1(out) -> voltage_FF/1(a)
  param/1 -> control_ab/2(param), Bus Selector/1
  I_ab_ref/1 -> Subtract1/1
  Voltage_lim/1(ab_out) -> Subtract/2, Divide/1

== system cascaded_droop_vi/cascaded/Subsystem4/voltage ==
  param : Inport
  U_ab_ref : Inport  Port=2
  U_ab : Inport  Port=3
  Ig_ab : Inport  Port=4
  Bus Selector : BusSelector  OutputSignals=g_ff_i,Isat
  Current_lim : Subsystem
  Delay : Delay  DelayLength=1  InitialCondition=0
  Subtract : Sum  Inputs=+-
  Subtract1 : Sum  Inputs=+-
  control_ab : Subsystem
  current_FF : Subsystem
  I_ab_ref : Outport  VectorParamsAs1DForOutWhenUnconnected=off
  wires:
  Bus Selector/2 -> Current_lim/2(Isat)  "<Isat>"
  U_ab_ref/1 -> Subtract1/1
  param/1 -> Bus Selector/1, control_ab/2(param)
  control_ab/1(out) -> current_FF/1(a)
  Subtract1/1 -> control_ab/1(in_ab)
  U_ab/1 -> Subtract1/2
  Bus Selector/1 -> current_FF/3(g_FF)  "<g_ff_i>"
  Subtract/1 -> Delay/1
  Ig_ab/1 -> current_FF/2(b)
  Current_lim/1(ab_out) -> I_ab_ref/1, Subtract/2
  Delay/1 -> control_ab/3(awr)
  current_FF/1(ab_out) -> Subtract/1, Current_lim/1(ab_in)

== system cascaded_droop_vi/cascaded controller/Subsystem1/Subsystem ==
  In1 : Inport
  Trigger : TriggerPort  VariantControl=Variant  PortDimensions=1
  Out1 : Outport  VectorParamsAs1DForOutWhenUnconnected=off
  wires:
  In1/1 -> Out1/1

== system cascaded_droop_vi/cascaded controller/cascaded/Cascaded Loop ==
  V_ref_dq0 : Inport
  I_inv_ab : Inport  Port=2
  theta : Inport  Port=3
  V_dc : Inport  Port=4
  param : Inport  Port=5
  V_cap_ab : Inport  Port=6
  ig_ab : Inport  Port=7
  Constant1 : Constant  Value=-2/9
  Scope : Scope
  Selector3 : Selector  IndexMode=Zero-based  InputPortWidth=3  IndexOptions=Index vector (dialog)  Indices=[0 1]  OutputSizes=1
  Subtract2 : Sum  Inputs=+-
  THI1 : Subsystem
  Virtual impedance : Subsystem
  alpha-beta to abc1 : Gain  Gain="[ 1   0; -1/2  sqrt(3)/2; -1/2  -sqrt(3)/2]"  Multiplication=Matrix(K*u) (u vector)  SaturateOnIntegerOverflow=on  OutDataTypeStr=Inherit: Same as input  ParamDataTypeStr=Inherit: Same as input
  current : Subsystem  VariantControl=PR
  dq0 to Alpha-Beta-Zero : spsdq0toAlphaBetaZeroLib/dq0 to Alpha-Beta-Zero  Alignment=90 degrees behind phase A axis
  voltage : Subsystem  VariantControl=PR
  MOD_PWM1 : Outport  VectorParamsAs1DForOutWhenUnconnected=off
  wires:
  dq0 to Alpha-Beta-Zero/1 -> Selector3/1
  V_ref_dq0/1 -> dq0 to Alpha-Beta-Zero/1
  Constant1/1 -> THI1/1(THI gain)
  THI1/1(abc_out) -> MOD_PWM1/1
  V_cap_ab/1 -> voltage/3(U_ab), current/4(U_ab)
  ig_ab/1 -> voltage/4(Ig_ab), Virtual impedance/1(Ig_ab)
  param/1 -> current/1(param), voltage/1(param)
  voltage/1(I_ab_ref) -> current/2(I_ab_ref)
  Subtract2/1 -> voltage/2(U_ab_ref)
  alpha-beta to abc1/1 -> THI1/2(abc)
  current/1(U_ab_inv) -> THI1/3(ab), alpha-beta to abc1/1
  Virtual impedance/1(U_Lv_ab) -> Subtract2/2
  V_dc/1 -> current/5(Udc)
  Selector3/1 -> Scope/1, Subtract2/1
  I_inv_ab/1 -> current/3(I_ab)
  theta/1 -> dq0 to Alpha-Beta-Zero/2

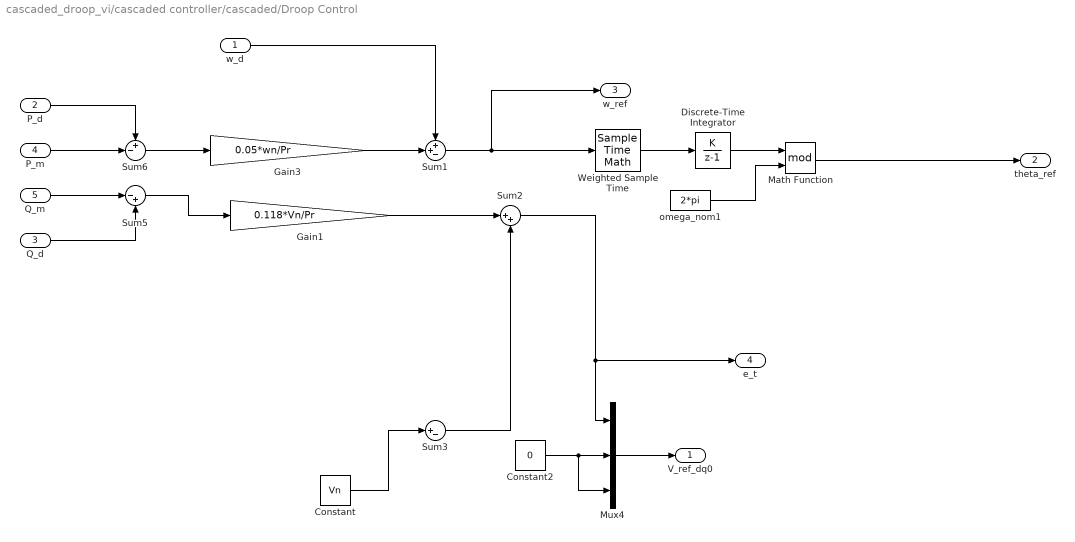
== system cascaded_droop_vi/cascaded controller/cascaded/Droop Control ==
  w_d : Inport
  P_d : Inport  Port=2
  Q_d : Inport  Port=3
  P_m : Inport  Port=4
  Q_m : Inport  Port=5
  Constant : Constant  Value=Vn
  Constant2 : Constant  Value=0
  Discrete-Time Integrator : DiscreteIntegrator  IntegratorMethod=Accumulation: Forward Euler  InitialCondition=pi*0  SampleTime=-1  ICPrevOutput=DiscIntNeverNeededParam  ICPrevScaledInput=DiscIntNeverNeededParam
  Gain1 : Gain  Gain=0.118*Vn/Pr
  Gain3 : Gain  Gain=0.05*wn/Pr
  Math Function : Math  Operator=mod  SignedPower=on  SaturateOnIntegerOverflow=on
  Mux4 : Mux  Inputs=3
  Sum1 : Sum  Inputs=++-
  Sum2 : Sum  Inputs=|++
  Sum3 : Sum  Inputs=|+-
  Sum5 : Sum  Inputs=|-+
  Sum6 : Sum  Inputs=+-|
  Weighted Sample Time : SampleTimeMath  TsampMathOp=*  TsampMathImp=Offline Scaling Adjustment
  omega_nom1 : Constant  Value=2*pi
  V_ref_dq0 : Outport
  theta_ref : Outport  Port=2
  w_ref : Outport  Port=3
  e_t : Outport  Port=4
  wires:
  Q_d/1 -> Sum5/2
  P_d/1 -> Sum6/1
  P_m/1 -> Sum6/2
  Q_m/1 -> Sum5/1
  Sum5/1 -> Gain1/1
  w_d/1 -> Sum1/1
  Sum3/1 -> Sum2/2
  Constant2/1 -> Mux4/3, Mux4/2
  Sum1/1 -> Weighted Sample Time/1, w_ref/1
  Mux4/1 -> V_ref_dq0/1
  Gain1/1 -> Sum2/1
  Constant/1 -> Sum3/1
  Sum2/1 -> Mux4/1, e_t/1
  Math Function/1 -> theta_ref/1
  omega_nom1/1 -> Math Function/2
  Discrete-Time Integrator/1 -> Math Function/1
  Weighted Sample Time/1 -> Discrete-Time Integrator/1
  Sum6/1 -> Gain3/1
  Gain3/1 -> Sum1/2

== system cascaded_droop_vi/cascaded controller/cascaded/Pythagoras ==
  ab : Inport
  Sqrt : Sqrt  SaturateOnIntegerOverflow=on
  Square : Math  Operator=square  SignedPower=on  RndMeth=Zero  SaturateOnIntegerOverflow=on
  Sum of Elements : Sum  Inputs=+
  magnitude : Outport  VectorParamsAs1DForOutWhenUnconnected=off
  wires:
  Sqrt/1 -> magnitude/1
  ab/1 -> Square/1
  Square/1 -> Sum of Elements/1
  Sum of Elements/1 -> Sqrt/1

== system cascaded_droop_vi/cascaded controller/cascaded/Subsystem ==
  1/kp_i : Constant  Value=1/Kpc_1
  1/kp_u : Constant  Value=1/kp_u
  Bus Creator : BusCreator  Inputs=11
  E1 : Constant  Value=wn*Lf_1
  E2 : Constant  Value=Cf_1*wn
  Isat : Constant  Value=Ilim
  g_ff_i : Constant
  g_ff_v : Constant
  ki_i*Ts/2 : Constant  Value=Kic_1
  ki_u*Ts/2 : Constant  Value=ki_u
  kp_i : Constant  Value=Kpc_1
  kp_u : Constant  Value=kp_u
  param : Outport  VectorParamsAs1DForOutWhenUnconnected=off
  wires:
  Bus Creator/1 -> param/1
  g_ff_v/1 -> Bus Creator/11  "g_ff_v"
  g_ff_i/1 -> Bus Creator/10  "g_ff_i"
  Isat/1 -> Bus Creator/9  "Isat"
  E2/1 -> Bus Creator/8  "E2"
  1/kp_u/1 -> Bus Creator/7  "1/kp_u"
  ki_u*Ts/2/1 -> Bus Creator/6  "ki_u"
  kp_u/1 -> Bus Creator/5  "kp_u"
  E1/1 -> Bus Creator/4  "E1"
  1/kp_i/1 -> Bus Creator/3  "1/kp_i"
  ki_i*Ts/2/1 -> Bus Creator/2  "ki_i"
  kp_i/1 -> Bus Creator/1  "kp_i"

== system cascaded_droop_vi/cascaded controller/cascaded/power calculation grid side ==
  voltage ab : Inport
  current ab : Inport  Port=2
  Demux : Demux  Outputs=2
  Demux1 : Demux  Outputs=2
  Gain1 : Gain  Gain=3/2
  Gain3 : Gain  Gain=3/2
  Product{1,4..6} (4 alike) : Product  InputSameDT=on  SaturateOnIntegerOverflow=on  OutDataTypeStr=Inherit: Same as first input
  Sum2 : Sum  Inputs=+-
  Sum3 : Sum
  abc to alpha-beta3 : Subsystem
  active power : Outport
  reactive power : Outport  Port=2
  wires:
  Product6/1 -> Sum2/2
  Product1/1 -> Sum2/1
  Sum2/1 -> Gain1/1
  Gain3/1 -> active power/1
  Product5/1 -> Sum3/2
  Demux1/2 -> Product5/2, Product6/2
  Demux/2 -> Product5/1, Product1/1
  Product4/1 -> Sum3/1
  Demux1/1 -> Product4/2, Product1/2
  Demux/1 -> Product6/1, Product4/1
  Sum3/1 -> Gain3/1
  Gain1/1 -> reactive power/1
  current ab/1 -> Demux1/1
  voltage ab/1 -> Demux/1

== system cascaded_droop_vi/cascaded/Subsystem4/current/Voltage_lim ==
  ab_in : Inport
  Vdc : Inport  Port=2
  Divide : Product  Inputs=*/
  Divide1 : Product  Inputs=**
  Gain : Gain  Gain=1/sqrt(3)
  Subsystem : Subsystem
  pythagoras : Subsystem
  ab_out : Outport  VectorParamsAs1DForOutWhenUnconnected=off
  wires:
  Gain/1 -> Divide/1, Subsystem/2(b)
  ab_in/1 -> Divide1/2, pythagoras/1(ab)
  pythagoras/1(|ab|) -> Subsystem/1(a)
  Vdc/1 -> Gain/1
  Subsystem/1(max) -> Divide/2
  Divide/1 -> Divide1/1
  Divide1/1 -> ab_out/1

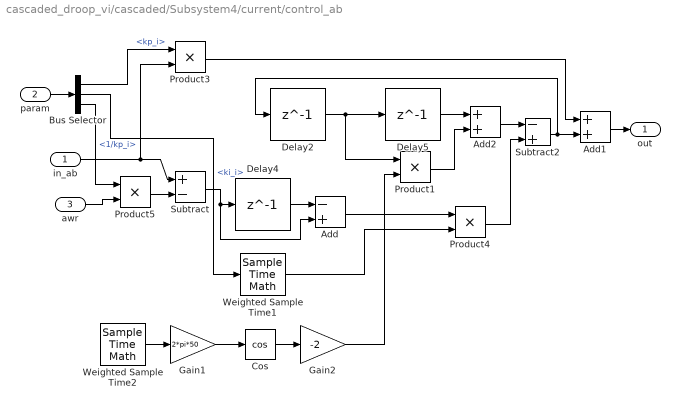
== system cascaded_droop_vi/cascaded/Subsystem4/current/control_ab ==
  in_ab : Inport
  param : Inport  Port=2
  awr : Inport  Port=3
  Add : Sum  Inputs=-+  AccumDataTypeStr=single
  Add1 : Sum
  Add2 : Sum
  Bus Selector : BusSelector  OutputSignals=kp_i,ki_i,1/kp_i
  Cos : Trigonometry  Operator=cos
  Delay2 : Delay  DelayLength=1  InitialCondition=0
  Delay4 : Delay  DelayLength=1  InitialCondition=0
  Delay5 : Delay  DelayLength=1  InitialCondition=0
  Gain1 : Gain  Gain=2*pi*50
  Gain2 : Gain  Gain=-2
  Product{1,3..5} (4 alike) : Product
  Subtract : Sum  Inputs=+-
  Subtract2 : Sum  Inputs=-+
  Weighted Sample Time1 : SampleTimeMath  TsampMathOp=*
  Weighted Sample Time2 : SampleTimeMath  TsampMathOp=Ts Only
  out : Outport  VectorParamsAs1DForOutWhenUnconnected=off
  wires:
  param/1 -> Bus Selector/1
  Product1/1 -> Add2/2
  Add1/1 -> out/1
  Product4/1 -> Subtract2/2
  Delay4/1 -> Add/1
  Subtract/1 -> Delay4/1, Add/2
  Add/1 -> Product4/1
  in_ab/1 -> Product3/2, Subtract/1
  Delay5/1 -> Add2/1
  Subtract2/1 -> Delay2/1, Add1/2
  Delay2/1 -> Product1/1, Delay5/1
  Add2/1 -> Subtract2/1
  Product3/1 -> Add1/1
  Bus Selector/1 -> Product3/1  "<kp_i>"
  Bus Selector/2 -> Weighted Sample Time1/1  "<ki_i>"
  Weighted Sample Time1/1 -> Product4/2
  Product5/1 -> Subtract/2
  awr/1 -> Product5/2
  Bus Selector/3 -> Product5/1  "<1/kp_i>"
  Weighted Sample Time2/1 -> Gain1/1
  Gain1/1 -> Cos/1
  Cos/1 -> Gain2/1
  Gain2/1 -> Product1/2

== system cascaded_droop_vi/cascaded/Subsystem4/current/voltage_FF ==
  a : Inport
  b : Inport  Port=2
  g_FF : Inport  Port=3
  Add5 : Sum
  Product : Product
  ab_out : Outport  VectorParamsAs1DForOutWhenUnconnected=off
  wires:
  Product/1 -> Add5/2
  b/1 -> Product/1
  g_FF/1 -> Product/2
  a/1 -> Add5/1
  Add5/1 -> ab_out/1

== system cascaded_droop_vi/cascaded/Subsystem4/voltage/Current_lim ==
  ab_in : Inport
  Isat : Inport  Port=2
  Divide : Product  Inputs=*/
  Divide1 : Product  Inputs=**
  Subsystem : Subsystem
  pythagoras : Subsystem
  ab_out : Outport  VectorParamsAs1DForOutWhenUnconnected=off
  wires:
  Divide1/1 -> ab_out/1
  Divide/1 -> Divide1/1
  Subsystem/1(max) -> Divide/2
  pythagoras/1(|ab|) -> Subsystem/1(a)
  ab_in/1 -> pythagoras/1(ab), Divide1/2
  Isat/1 -> Subsystem/2(b), Divide/1
